simulink model "inference_task"  (Simulink 3.00)
libraries: logiclib x16, langlib x8, genlib x1
settings Model: MaskType=REX sequence  MaskIconFrame=on  MaskIconOpaque=on  MaskIconRotate=none  MaskIconUnits=autoscale

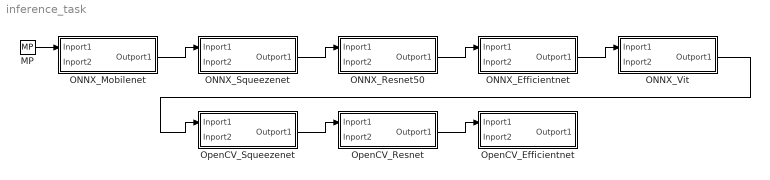
== system inference_task ==
  MP : genlib/MP  BSTATE=off  pwidth=1  RPTF=off
  ONNX_Efficientnet : Subsystem
      mask Type: REX sequence
  ONNX_Mobilenet : Subsystem
      mask Type: REX sequence
  ONNX_Resnet50 : Subsystem
      mask Type: REX sequence
  ONNX_Squeezenet : Subsystem
      mask Type: REX sequence
  ONNX_Vit : Subsystem
      mask Type: REX sequence
  OpenCV_Efficientnet : Subsystem
      mask Type: REX sequence
  OpenCV_Resnet : Subsystem
      mask Type: REX sequence
  OpenCV_Squeezenet : Subsystem
      mask Type: REX sequence
  wires:
  MP/1 -> ONNX_Mobilenet/1(Inport1)
  ONNX_Efficientnet/1(Outport1) -> ONNX_Vit/1(Inport1)
  ONNX_Mobilenet/1(Outport1) -> ONNX_Squeezenet/1(Inport1)
  ONNX_Resnet50/1(Outport1) -> ONNX_Efficientnet/1(Inport1)
  ONNX_Squeezenet/1(Outport1) -> ONNX_Resnet50/1(Inport1)
  ONNX_Vit/1(Outport1) -> OpenCV_Squeezenet/1(Inport1)
  OpenCV_Resnet/1(Outport1) -> OpenCV_Efficientnet/1(Inport1)
  OpenCV_Squeezenet/1(Outport1) -> OpenCV_Resnet/1(Inport1)

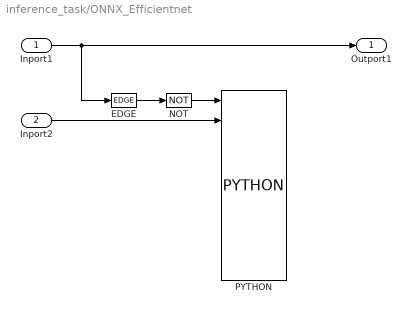
== system inference_task/ONNX_Efficientnet ==
  Inport1 : Inport  Port=1  OutDataTypeStr=Inherit: auto
  Inport2 : Inport  Port=2  OutDataTypeStr=Inherit: auto
  EDGE : logiclib/EDGE  iedge=1: Rising edge
  NOT : logiclib/NOT
  PYTHON : langlib/PYTHON  srcname=inference.py  embedded=on  p0=/mnt/external_hdd/InferenceRexTest  p1=efficientnet_b0  p2=onnxruntime
  Outport1 : Outport  Port=1  OutDataTypeStr=Inherit: auto
  wires:
  EDGE/1 -> NOT/1
  Inport1/1 -> EDGE/1, Outport1/1
  Inport2/1 -> PYTHON/3
  NOT/1 -> PYTHON/1

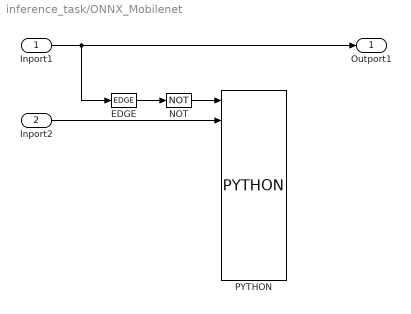
== system inference_task/ONNX_Mobilenet ==
  Inport1 : Inport  Port=1  OutDataTypeStr=Inherit: auto
  Inport2 : Inport  Port=2  OutDataTypeStr=Inherit: auto
  EDGE : logiclib/EDGE  iedge=1: Rising edge
  NOT : logiclib/NOT
  PYTHON : langlib/PYTHON  srcname=inference.py  embedded=on  p0=/mnt/external_hdd/InferenceRexTest  p1=mobilenetv2  p2=onnxruntime
  Outport1 : Outport  Port=1  OutDataTypeStr=Inherit: auto
  wires:
  EDGE/1 -> NOT/1
  Inport1/1 -> EDGE/1, Outport1/1
  Inport2/1 -> PYTHON/3
  NOT/1 -> PYTHON/1

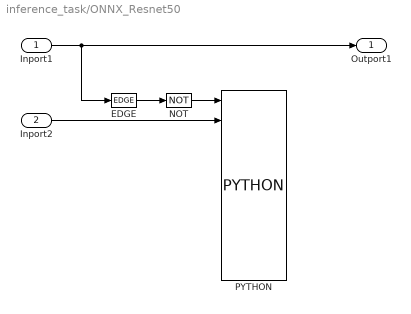
== system inference_task/ONNX_Resnet50 ==
  Inport1 : Inport  Port=1  OutDataTypeStr=Inherit: auto
  Inport2 : Inport  Port=2  OutDataTypeStr=Inherit: auto
  EDGE : logiclib/EDGE  iedge=1: Rising edge
  NOT : logiclib/NOT
  PYTHON : langlib/PYTHON  srcname=inference.py  embedded=on  p0=/mnt/external_hdd/InferenceRexTest  p1=resnet50  p2=onnxruntime
  Outport1 : Outport  Port=1  OutDataTypeStr=Inherit: auto
  wires:
  EDGE/1 -> NOT/1
  Inport1/1 -> EDGE/1, Outport1/1
  Inport2/1 -> PYTHON/3
  NOT/1 -> PYTHON/1

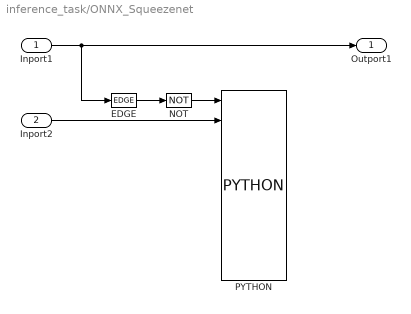
== system inference_task/ONNX_Squeezenet ==
  Inport1 : Inport  Port=1  OutDataTypeStr=Inherit: auto
  Inport2 : Inport  Port=2  OutDataTypeStr=Inherit: auto
  EDGE : logiclib/EDGE  iedge=1: Rising edge
  NOT : logiclib/NOT
  PYTHON : langlib/PYTHON  srcname=inference.py  embedded=on  p0=/mnt/external_hdd/InferenceRexTest  p1=squeezenet  p2=onnxruntime
  Outport1 : Outport  Port=1  OutDataTypeStr=Inherit: auto
  wires:
  EDGE/1 -> NOT/1
  Inport1/1 -> EDGE/1, Outport1/1
  Inport2/1 -> PYTHON/3
  NOT/1 -> PYTHON/1

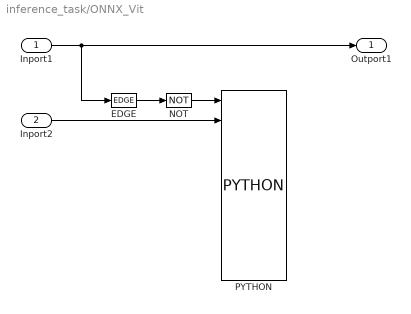
== system inference_task/ONNX_Vit ==
  Inport1 : Inport  Port=1  OutDataTypeStr=Inherit: auto
  Inport2 : Inport  Port=2  OutDataTypeStr=Inherit: auto
  EDGE : logiclib/EDGE  iedge=1: Rising edge
  NOT : logiclib/NOT
  PYTHON : langlib/PYTHON  srcname=inference.py  embedded=on  p0=/mnt/external_hdd/InferenceRexTest  p1=vit_b16  p2=onnxruntime
  Outport1 : Outport  Port=1  OutDataTypeStr=Inherit: auto
  wires:
  EDGE/1 -> NOT/1
  Inport1/1 -> EDGE/1, Outport1/1
  Inport2/1 -> PYTHON/3
  NOT/1 -> PYTHON/1

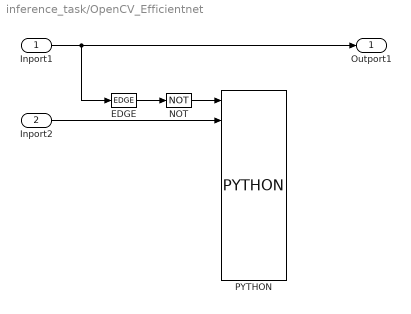
== system inference_task/OpenCV_Efficientnet ==
  Inport1 : Inport  Port=1  OutDataTypeStr=Inherit: auto
  Inport2 : Inport  Port=2  OutDataTypeStr=Inherit: auto
  EDGE : logiclib/EDGE  iedge=1: Rising edge
  NOT : logiclib/NOT
  PYTHON : langlib/PYTHON  srcname=inference.py  embedded=on  p0=/mnt/external_hdd/InferenceRexTest  p1=efficientnet_b0  p2=opencv
  Outport1 : Outport  Port=1  OutDataTypeStr=Inherit: auto
  wires:
  EDGE/1 -> NOT/1
  Inport1/1 -> EDGE/1, Outport1/1
  Inport2/1 -> PYTHON/3
  NOT/1 -> PYTHON/1

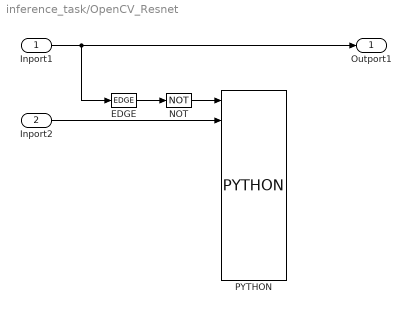
== system inference_task/OpenCV_Resnet ==
  Inport1 : Inport  Port=1  OutDataTypeStr=Inherit: auto
  Inport2 : Inport  Port=2  OutDataTypeStr=Inherit: auto
  EDGE : logiclib/EDGE  iedge=1: Rising edge
  NOT : logiclib/NOT
  PYTHON : langlib/PYTHON  srcname=inference.py  embedded=on  p0=/mnt/external_hdd/InferenceRexTest  p1=resnet50  p2=opencv
  Outport1 : Outport  Port=1  OutDataTypeStr=Inherit: auto
  wires:
  EDGE/1 -> NOT/1
  Inport1/1 -> EDGE/1, Outport1/1
  Inport2/1 -> PYTHON/3
  NOT/1 -> PYTHON/1

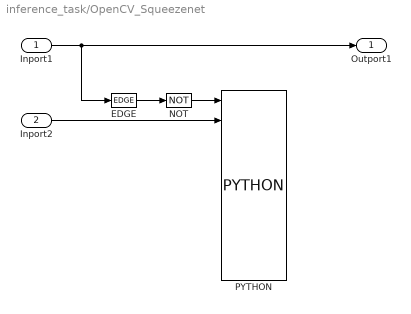
== system inference_task/OpenCV_Squeezenet ==
  Inport1 : Inport  Port=1  OutDataTypeStr=Inherit: auto
  Inport2 : Inport  Port=2  OutDataTypeStr=Inherit: auto
  EDGE : logiclib/EDGE  iedge=1: Rising edge
  NOT : logiclib/NOT
  PYTHON : langlib/PYTHON  srcname=inference.py  embedded=on  p0=/mnt/external_hdd/InferenceRexTest  p1=squeezenet  p2=opencv
  Outport1 : Outport  Port=1  OutDataTypeStr=Inherit: auto
  wires:
  EDGE/1 -> NOT/1
  Inport1/1 -> EDGE/1, Outport1/1
  Inport2/1 -> PYTHON/3
  NOT/1 -> PYTHON/1
